simulink model "batteriemodell_simscape_2output"  (R2024a)
settings: Solver=FixedStepAuto  StartTime=0.0  StopTime=10000  RelTol=1e-3
libraries: fl_lib x27, nesl_utility x15
settings Model: ExtModeTrigDuration=100  Creator=lenna  LastModifiedBy=lenna
settings DataIOCC: StateSaveName=tmp_raccel_xout
settings OptimizationCC: EfficientMapNaN2IntZero=off
settings DebuggingCC: ModelReferenceSymbolNameMessage=none
settings HardwareCC: TargetBitPerPointer=64  TargetBitPerSizeT=64  TargetBitPerPtrDiffT=64  TargetLongLongMode=on  TargetIntDivRoundTo=Zero  TargetEndianess=LittleEndian  TargetWordSize=64  TargetHWDeviceType=MATLAB Host  ProdEqTarget=off
settings RTWCC: Description=FMU based on GRT (Functional Mock-up Unit)  SystemTargetFile=grtfmi.tlc  GenerateMakefile=off  TemplateMakefile=none  RTWVerbose=off  RetainRTWFile=on  RTWUseSimCustomCode=on  CustomBLASCallback=coder.internal.blas.MATLABBLASCallback
settings CodeAppCC: GenerateComments=off  MaxIdLength=128  SimulinkBlockComments=off
settings STFCustomTargetCC: CombineOutputUpdateFcns=on  GRTInterface=off  UseToolchainInfoCompliant=off  SystemTargetFile=grtfmi.tlc
settings GRTTargetCC: ParMdlRefBuildCompliant=off  CompOptLevelCompliant=off  ConcurrentExecutionCompliant=off  MatFileLogging=off  CPPClassGenCompliant=off  UseToolchainInfoCompliant=off

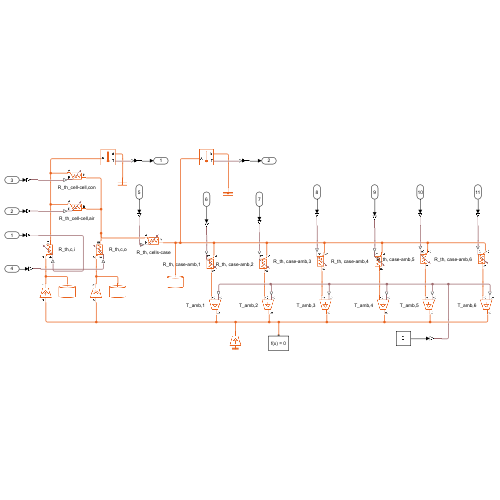
[thumbnail: Simulink's stored preview of the top-level diagram]
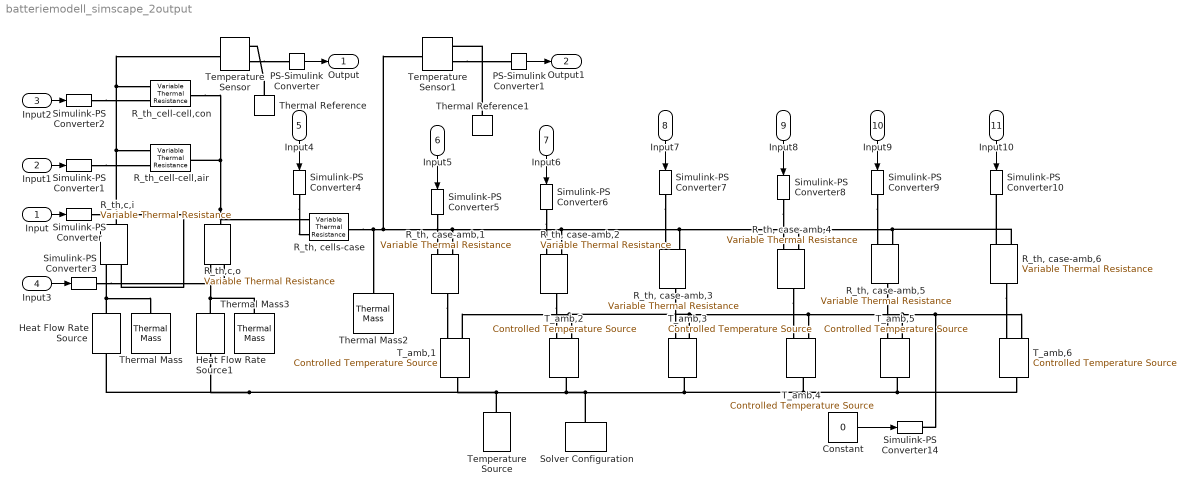
== system batteriemodell_simscape_2output ==
  Input : Inport
  Input1 : Inport  Port=2
  Input2 : Inport  Port=3
  Input3 : Inport  Port=4
  Input4 : Inport  Port=5
  Input5 : Inport  Port=6
  Input6 : Inport  Port=7
  Input7 : Inport  Port=8
  Input8 : Inport  Port=9
  Input9 : Inport  Port=10
  Input10 : Inport  Port=11
  Constant : Constant  Value=0
  Heat Flow Rate Source : fl_lib/Thermal/Thermal Sources/Heat Flow Rate Source  heat_flow=10 W
      settings: InternalSimscapePortConfiguration="{\"Bottom\":[],\"Left\":[{\"id\":\"B\",\"label\":\"B\",\"type\":\"foundation.thermal.thermal\"}],\"Right\":[{\"id\":\"A\",\"label\":\"A\",\"type\":\"foundation.thermal.thermal\"}],\"Top\":[]}"
  Heat Flow Rate Source1 : fl_lib/Thermal/Thermal Sources/Heat Flow Rate Source  heat_flow=10 W
      settings: InternalSimscapePortConfiguration="{\"Bottom\":[],\"Left\":[{\"id\":\"B\",\"label\":\"B\",\"type\":\"foundation.thermal.thermal\"}],\"Right\":[{\"id\":\"A\",\"label\":\"A\",\"type\":\"foundation.thermal.thermal\"}],\"Top\":[]}"
  PS-Simulink Converter : nesl_utility/PS-Simulink Converter  PhysicalDomain=network_engine_domain  SubClassName=ps_output  LeftPortType=input  RightPortType=output  PseudoPeriodic=off  Frequencies=[]  VectorFormat=inherit  Unit=inherit  AffineConversion=off
  PS-Simulink Converter1 : nesl_utility/PS-Simulink Converter  PhysicalDomain=network_engine_domain  SubClassName=ps_output  LeftPortType=input  RightPortType=output  PseudoPeriodic=off  Frequencies=[]  VectorFormat=inherit  Unit=inherit  AffineConversion=off
  R_th, case-amb,{1..6} (6 alike) : fl_lib/Thermal/Thermal Elements/Variable Thermal Resistance  R_min=0 K/W  T_specify=off  T_priority=None  T=0 K  T_nominal_specify=off  T_nominal_value=1  T_nominal_unit=K  Q_specify=off  Q_priority=None  Q=0 W  Q_nominal_specify=off  Q_nominal_value=1  Q_nominal_unit=W
      settings: InternalSimscapePortConfiguration="{\"Bottom\":[],\"Left\":[{\"id\":\"A\",\"label\":\"A\",\"type\":\"foundation.thermal.thermal\"},{\"id\":\"R\",\"label\":\"R\",\"type\":\"input\"}],\"Right\":[{\"id\":\"B\",\"label\":\"B\",\"type\":\"foundation.thermal.thermal\"}],\"Top\":[]}"
  "R_th, cells-case" : fl_lib/Thermal/Thermal Elements/Variable Thermal Resistance  R_min=0 K/W  T_specify=off  T_priority=None  T=0 K  T_nominal_specify=off  T_nominal_value=1  T_nominal_unit=K  Q_specify=off  Q_priority=None  Q=0 W  Q_nominal_specify=off  Q_nominal_value=1  Q_nominal_unit=W
      settings: InternalSimscapePortConfiguration="{\"Bottom\":[],\"Left\":[{\"id\":\"A\",\"label\":\"A\",\"type\":\"foundation.thermal.thermal\"},{\"id\":\"R\",\"label\":\"R\",\"type\":\"input\"}],\"Right\":[{\"id\":\"B\",\"label\":\"B\",\"type\":\"foundation.thermal.thermal\"}],\"Top\":[]}"
  R_th,c,i : fl_lib/Thermal/Thermal Elements/Variable Thermal Resistance  R_min=0 K/W  T_specify=off  T_priority=None  T=0 K  T_nominal_specify=off  T_nominal_value=1  T_nominal_unit=K  Q_specify=off  Q_priority=None  Q=0 W  Q_nominal_specify=off  Q_nominal_value=1  Q_nominal_unit=W
      settings: InternalSimscapePortConfiguration="{\"Bottom\":[],\"Left\":[{\"id\":\"A\",\"label\":\"A\",\"type\":\"foundation.thermal.thermal\"},{\"id\":\"R\",\"label\":\"R\",\"type\":\"input\"}],\"Right\":[{\"id\":\"B\",\"label\":\"B\",\"type\":\"foundation.thermal.thermal\"}],\"Top\":[]}"
  R_th,c,o : fl_lib/Thermal/Thermal Elements/Variable Thermal Resistance  R_min=0 K/W  T_specify=off  T_priority=None  T=0 K  T_nominal_specify=off  T_nominal_value=1  T_nominal_unit=K  Q_specify=off  Q_priority=None  Q=0 W  Q_nominal_specify=off  Q_nominal_value=1  Q_nominal_unit=W
      settings: InternalSimscapePortConfiguration="{\"Bottom\":[],\"Left\":[{\"id\":\"A\",\"label\":\"A\",\"type\":\"foundation.thermal.thermal\"},{\"id\":\"R\",\"label\":\"R\",\"type\":\"input\"}],\"Right\":[{\"id\":\"B\",\"label\":\"B\",\"type\":\"foundation.thermal.thermal\"}],\"Top\":[]}"
  R_th_cell-cell,air : fl_lib/Thermal/Thermal Elements/Variable Thermal Resistance  R_min=0 K/W  T_specify=off  T_priority=None  T=0 K  T_nominal_specify=off  T_nominal_value=1  T_nominal_unit=K  Q_specify=off  Q_priority=None  Q=0 W  Q_nominal_specify=off  Q_nominal_value=1  Q_nominal_unit=W
      settings: InternalSimscapePortConfiguration="{\"Bottom\":[],\"Left\":[{\"id\":\"A\",\"label\":\"A\",\"type\":\"foundation.thermal.thermal\"},{\"id\":\"R\",\"label\":\"R\",\"type\":\"input\"}],\"Right\":[{\"id\":\"B\",\"label\":\"B\",\"type\":\"foundation.thermal.thermal\"}],\"Top\":[]}"
  R_th_cell-cell,con : fl_lib/Thermal/Thermal Elements/Variable Thermal Resistance  R_min=0 K/W  T_specify=off  T_priority=None  T=0 K  T_nominal_specify=off  T_nominal_value=1  T_nominal_unit=K  Q_specify=off  Q_priority=None  Q=0 W  Q_nominal_specify=off  Q_nominal_value=1  Q_nominal_unit=W
      settings: InternalSimscapePortConfiguration="{\"Bottom\":[],\"Left\":[{\"id\":\"A\",\"label\":\"A\",\"type\":\"foundation.thermal.thermal\"},{\"id\":\"R\",\"label\":\"R\",\"type\":\"input\"}],\"Right\":[{\"id\":\"B\",\"label\":\"B\",\"type\":\"foundation.thermal.thermal\"}],\"Top\":[]}"
  Simulink-PS Converter{,1..10,14} (12 alike) : nesl_utility/Simulink-PS Converter  PhysicalDomain=network_engine_domain  SubClassName=ps_input  LeftPortType=input  RightPortType=output  PseudoPeriodic=off  Frequencies=[]  NoiseDistribution=none  NoiseParameters=[]  Unit=1  AffineConversion=off  FilteringAndDerivatives=provide  SimscapeFilterOrder=1  InputFilterTimeConstant=0.001  UdotUserProvided=0
  Solver Configuration : nesl_utility/Solver Configuration  PhysicalDomain=network_engine_domain  SubClassName=solver  LeftPortType=input  RightPortType=generic  Tones=[]  Harmonics=[]  SimulateNoise=off  Profile=off  UseLocalSampling=off  EnableSwitchedLinearOptims=on  FrequencyDomain=off  UseCCode=off  RelTol=0.001  AbsTol=0.001  MinStep=1e-09  ToWorkspace=off  RevertToSquareIcSolve=off  NumHomotopyIterations=100  PhasorMode=off  PhasorModeNumHarmonics=1  ConsistencySolver=NEWTON_XTOL_AFTER_FTOL  IndexReductionMethod=DerivativeReplacement  DoDC=off  ResidualTolerance=1e-09  ConsistencyTolSource=GLOBAL  ConsistencyAbsTol=0.001  ConsistencyRelTol=0.001  ConsistencyTolFactor=0.001  UseLocalSolver=off  LocalSolverChoice=NE_BACKWARD_EULER_ADVANCER  ResolveIndetEquations=on  FunctionEvalNumThread=1  LocalSolverSampleTime=0.001  DoFixedCost=off  MaxNonlinIter=3  MaxModeIter=2  ComputeImpulses=off  ImpulseIterations=2  LinearAlgebra=auto  LinearAlgebraNumThread=0  EquationFormulation=NE_TIME_EF  DelaysMemoryBudget=1024  AutomaticFiltering=on  FilteringTimeConstant=0.001  PartitionStorageMethod=AS_NEEDED  PartitionMemoryBudget=1024  PartitionMethod=ROBUST  MultibodyUseLocalSolver=off  MultibodyLocalSolverChoice=ODE1  MultibodyLocalSolverSampleTime=0.001
  T_amb,{1..6} (6 alike) : fl_lib/Thermal/Thermal Sources/Controlled Temperature Source
  Temperature Sensor : fl_lib/Thermal/Thermal Sensors/Temperature Sensor  temperature_measure=foundation.enum.MeasurementReference.difference
  Temperature Sensor1 : fl_lib/Thermal/Thermal Sensors/Temperature Sensor  temperature_measure=foundation.enum.MeasurementReference.difference
  Temperature Source : fl_lib/Thermal/Thermal Sources/Temperature Source  temperature=294.15 K
  Thermal Mass : fl_lib/Thermal/Thermal Elements/Thermal Mass  mass_type=foundation.enum.constant_variable.constant  mass=7*22*0.0438 kg  sp_heat=34.932/0.0438 J/(K*kg)  mass_min=1e-6 kg  num_ports=foundation.enum.numPorts2.one  m_specify=off  m_priority=High  m=1 kg  m_nominal_specify=off  m_nominal_value=1  m_nominal_unit=kg  T_specify=on  T_priority=High  T=294.15 K  T_nominal_specify=off  T_nominal_value=294.15  T_nominal_unit=K  Q_specify=off  Q_priority=None  Q=0 W  Q_nominal_specify=off  Q_nominal_value=1  Q_nominal_unit=W
  Thermal Mass2 : fl_lib/Thermal/Thermal Elements/Thermal Mass  mass_type=foundation.enum.constant_variable.constant  mass=0.2 kg  sp_heat=550 J/(K*kg)  mass_min=1e-6 kg  num_ports=foundation.enum.numPorts2.one  m_specify=off  m_priority=High  m=1 kg  m_nominal_specify=off  m_nominal_value=1  m_nominal_unit=kg  T_specify=on  T_priority=High  T=294.15 K  T_nominal_specify=off  T_nominal_value=294.15  T_nominal_unit=K  Q_specify=off  Q_priority=None  Q=0 W  Q_nominal_specify=off  Q_nominal_value=1  Q_nominal_unit=W
  Thermal Mass3 : fl_lib/Thermal/Thermal Elements/Thermal Mass  mass_type=foundation.enum.constant_variable.constant  mass=7*22*0.0438 kg  sp_heat=34.932/0.0438 J/(K*kg)  mass_min=1e-6 kg  num_ports=foundation.enum.numPorts2.one  m_specify=off  m_priority=High  m=1 kg  m_nominal_specify=off  m_nominal_value=1  m_nominal_unit=kg  T_specify=on  T_priority=High  T=294.15 K  T_nominal_specify=off  T_nominal_value=294.15  T_nominal_unit=K  Q_specify=off  Q_priority=None  Q=0 W  Q_nominal_specify=off  Q_nominal_value=1  Q_nominal_unit=W
  Thermal Reference : fl_lib/Thermal/Thermal Elements/Thermal Reference
  Thermal Reference1 : fl_lib/Thermal/Thermal Elements/Thermal Reference
  Output : Outport
  Output1 : Outport  Port=2
  wires:
  Input/1 -> Simulink-PS Converter/1
  PS-Simulink Converter/1 -> Output/1
  Input1/1 -> Simulink-PS Converter1/1
  Input2/1 -> Simulink-PS Converter2/1
  Input3/1 -> Simulink-PS Converter3/1
  Input4/1 -> Simulink-PS Converter4/1
  Input5/1 -> Simulink-PS Converter5/1
  Input6/1 -> Simulink-PS Converter6/1
  Input7/1 -> Simulink-PS Converter7/1
  Input8/1 -> Simulink-PS Converter8/1
  Input9/1 -> Simulink-PS Converter9/1
  Input10/1 -> Simulink-PS Converter10/1
  Constant/1 -> Simulink-PS Converter14/1
  PS-Simulink Converter1/1 -> Output1/1
  connections:
  Heat Flow Rate Source1/LConn1 -- Thermal Mass3/LConn1 -- R_th,c,o/LConn1
  R_th_cell-cell,con/RConn1 -- R_th_cell-cell,air/RConn1 -- "R_th, cells-case"/LConn1 -- R_th,c,o/RConn1
  "R_th, cells-case"/RConn1 -- "R_th, case-amb,6"/LConn1 -- "R_th, case-amb,5"/LConn1 -- "R_th, case-amb,4"/LConn1 -- "R_th, case-amb,3"/LConn1 -- "R_th, case-amb,2"/LConn1 -- "R_th, case-amb,1"/LConn1 -- Temperature Sensor1/LConn1 -- Thermal Mass2/LConn1
  "R_th, case-amb,6"/RConn1 -- T_amb,6/RConn2
  "R_th, case-amb,5"/RConn1 -- T_amb,5/RConn2
  "R_th, case-amb,2"/RConn1 -- T_amb,2/RConn2
  "R_th, case-amb,1"/RConn1 -- T_amb,1/RConn2
  "R_th, case-amb,4"/RConn1 -- T_amb,4/RConn2
  "R_th, case-amb,3"/RConn1 -- T_amb,3/RConn2
  Simulink-PS Converter/RConn1 -- R_th,c,i/LConn2
  Temperature Sensor/RConn2 -- PS-Simulink Converter/LConn1
  Simulink-PS Converter3/RConn1 -- R_th,c,o/LConn2
  Simulink-PS Converter4/RConn1 -- "R_th, cells-case"/LConn2
  Simulink-PS Converter5/RConn1 -- "R_th, case-amb,1"/LConn2
  Simulink-PS Converter6/RConn1 -- "R_th, case-amb,2"/LConn2
  Simulink-PS Converter7/RConn1 -- "R_th, case-amb,3"/LConn2
  Simulink-PS Converter8/RConn1 -- "R_th, case-amb,4"/LConn2
  Simulink-PS Converter9/RConn1 -- "R_th, case-amb,5"/LConn2
  "R_th, case-amb,6"/LConn2 -- Simulink-PS Converter10/RConn1
  Simulink-PS Converter2/RConn1 -- R_th_cell-cell,con/LConn2
  Simulink-PS Converter1/RConn1 -- R_th_cell-cell,air/LConn2
  T_amb,3/RConn1 -- T_amb,1/RConn1 -- T_amb,2/RConn1 -- T_amb,4/RConn1 -- T_amb,5/RConn1 -- Simulink-PS Converter14/RConn1 -- T_amb,6/RConn1
  Thermal Reference/LConn1 -- Temperature Sensor/RConn1
  Thermal Reference1/LConn1 -- Temperature Sensor1/RConn1
  Temperature Sensor1/RConn2 -- PS-Simulink Converter1/LConn1
  T_amb,6/LConn1 -- Temperature Source/LConn1 -- T_amb,1/LConn1 -- Heat Flow Rate Source/RConn1 -- Heat Flow Rate Source1/RConn1 -- T_amb,2/LConn1 -- Solver Configuration/RConn1 -- T_amb,3/LConn1 -- T_amb,4/LConn1 -- T_amb,5/LConn1
  Heat Flow Rate Source/LConn1 -- Thermal Mass/LConn1 -- R_th,c,i/LConn1
  R_th,c,i/RConn1 -- Temperature Sensor/LConn1 -- R_th_cell-cell,con/LConn1 -- R_th_cell-cell,air/LConn1
